simulink model "Discrete_SecondOrder_nonlinear"  (R2024a)
settings: Solver=FixedStepDiscrete  StartTime=0.0  StopTime=1  RelTol=1e-3
settings Model: Creator=perruquetti  LastModifiedBy=perruquetti

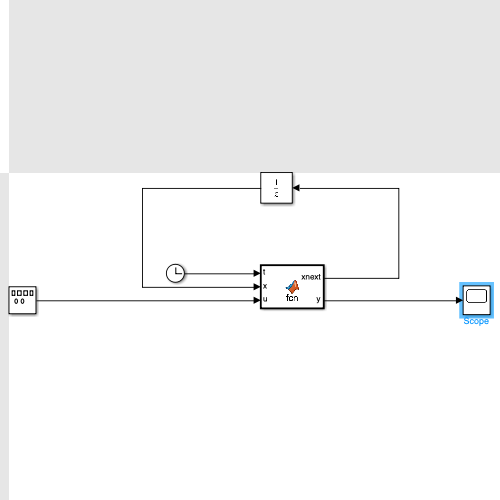
[thumbnail: Simulink's stored preview of the top-level diagram]
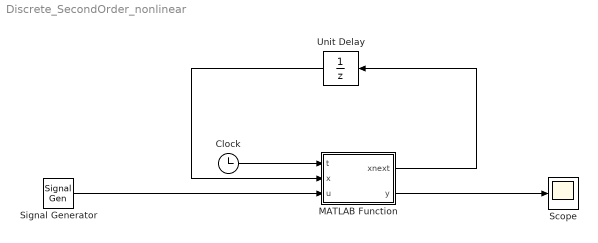
== system Discrete_SecondOrder_nonlinear ==
  Clock : Clock
  MATLAB Function : MATLAB Function  TreatAsAtomicUnit=on
  Scope : Scope
  Signal Generator : SignalGenerator  WaveForm=square  Amplitude=0.1  Units=rad/sec
  Unit Delay : UnitDelay  InitialCondition=[-0.12;0]  SampleTime=-1  HasFrameUpgradeWarning=on
  wires:
  MATLAB Function/1(xnext) -> Unit Delay/1
  Unit Delay/1 -> MATLAB Function/2(x)
  MATLAB Function/2(y) -> Scope/1
  Signal Generator/1 -> MATLAB Function/3(u)
  Clock/1 -> MATLAB Function/1(t)

== matlab function Discrete_SecondOrder_nonlinear/MATLAB Function ==
  data: t input; x input; xnext output; u input; y output
function [xnext,y] = fcn(t,x,u)
% constants
    a = 2;
%   x1 = -0.12; defined as external IC for the integrator
%   x2 = 0;     
% nonlinear set of equations
    xnext = [x(1)+0.1*(x(2)-cos(t)*x(1));
            x(2)+0.1*(a*x(1)-x(2)^3+sin(t)*u)];
    y = x';
